simulink model "chap4_3sim"  (Simulink 8.3)
settings: Solver=ode45  StartTime=0.0  StopTime=30  RelTol=1e-3
settings Model: Creator=liujk  LastModifiedBy=Prof_Liu  ExtModeTrigMode=oneshot  ExtModeArmWhenConnect=off
settings DataIOCC: LimitDataPoints=off  SignalLoggingName=sigsOut
settings OptimizationCC: BooleanDataType=off
settings DebuggingCC: SaveWithParameterizedLinksMsg=none  SignalResolutionControl=TryResolveAllWithWarning  SolverPrmCheckMsg=none  MultiTaskDSMMsg=warning  MultiTaskCondExecSysMsg=none
settings HardwareCC: TargetUnknown=on
settings RTWCC: IncludeERTFirstTime=on

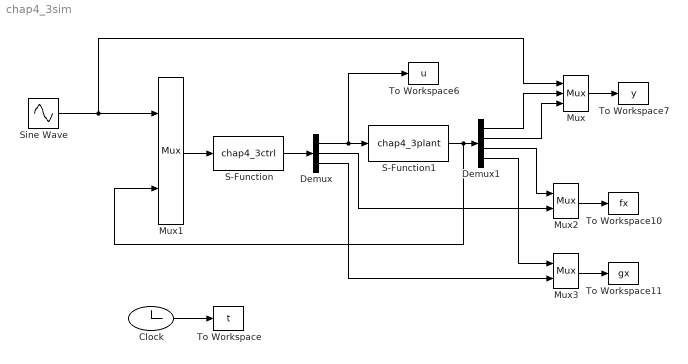
== system chap4_3sim ==
  Clock : Clock
  Demux : Demux  Outputs=3
  Demux1 : Demux
  Mux : Mux  Inputs=3
  Mux1 : Mux  Inputs=2
  Mux2 : Mux  Inputs=2
  Mux3 : Mux  Inputs=2
  S-Function : S-Function  FunctionName=chap4_3ctrl  EnableBusSupport=off
  S-Function1 : S-Function  FunctionName=chap4_3plant  EnableBusSupport=off
  Sine Wave : Sin  Amplitude=0.1  SampleTime=0
  To Workspace : ToWorkspace  VariableName=t  SampleTime=-1
  To Workspace10 : ToWorkspace  VariableName=fx  SampleTime=-1
  To Workspace11 : ToWorkspace  VariableName=gx  SampleTime=-1
  To Workspace6 : ToWorkspace  VariableName=u  SampleTime=-1
  To Workspace7 : ToWorkspace  VariableName=y  SampleTime=-1
  wires:
  Mux1/1 -> S-Function/1
  S-Function/1 -> Demux/1
  Sine Wave/1 -> Mux1/1, Mux/1
  S-Function1/1 -> Mux1/2, Demux1/1
  Demux/1 -> S-Function1/1, To Workspace6/1
  Clock/1 -> To Workspace/1
  Mux/1 -> To Workspace7/1
  Demux1/1 -> Mux/2
  Mux2/1 -> To Workspace10/1
  Demux/2 -> Mux2/2
  Mux3/1 -> To Workspace11/1
  Demux/3 -> Mux3/2
  Demux1/4 -> Mux3/1
  Demux1/3 -> Mux2/1
  Demux1/2 -> Mux/3
